simulink model "model_test"  (R2019b)
settings: Solver=VariableStepAuto  StartTime=0.0  StopTime=2000  RelTol=1e-3
values from neighbouring files (symbols this model uses):
  Belt_length = 0.5    [initialization.m]
  n = n+1    (= 2)    [training.m]
  num = 5    [initialization.m]    (also in training.m = 15)
undefined symbols (not defined in the file or in its folder): m, T_product
libraries: simulink x14, sldelib x14, rllib x4
settings Model: Creator=Alexa  LastModifiedBy=Alexa

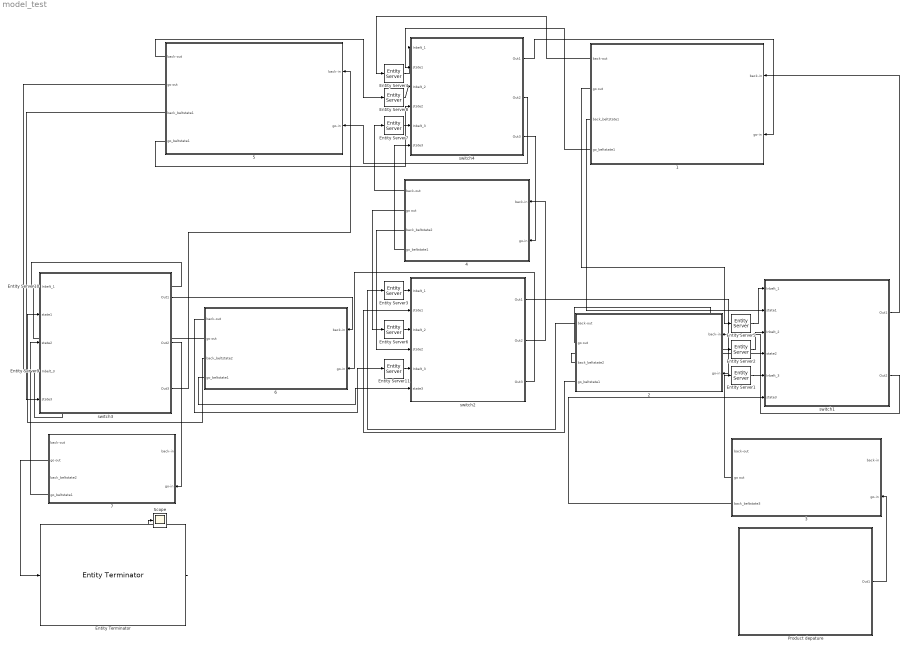
== system model_test ==
  "1 " : Subsystem
      mask Display: image('C:\Users\Alexa\Desktop\MA\writing\pic\thumbnail_image002.jpg'); % Use "Edit Image" on toolstrip to change.
  "2 " : Subsystem
      mask Display: image('C:\Users\Alexa\Desktop\MA\writing\pic\thumbnail_image010.png'); % Use "Edit Image" on toolstrip to change.
  "3 " : Subsystem
      mask Display: image('C:\Users\Alexa\Desktop\MA\writing\pic\thumbnail_image010.png'); % Use "Edit Image" on toolstrip to change.
  4 : Subsystem
      mask Display: image('C:\Users\Alexa\Desktop\MA\writing\pic\thumbnail_image010.png'); % Use "Edit Image" on toolstrip to change.
  5 : Subsystem
      mask Display: image('C:\Users\Alexa\Desktop\MA\writing\pic\thumbnail_image002.jpg'); % Use "Edit Image" on toolstrip to change.
  6 : Subsystem
      mask Display: image('C:\Users\Alexa\Desktop\MA\writing\pic\thumbnail_image010.png'); % Use "Edit Image" on toolstrip to change.
  7 : Subsystem
      mask Display: image('C:\Users\Alexa\Desktop\MA\writing\pic\thumbnail_image010.png'); % Use "Edit Image" on toolstrip to change.
  Entity Server{1,7,9,11} (4 alike) : EntityServer  InputPortMessageModes=m  OutputPortMessageModes=m  Capacity=1  ServiceTimeValue=0  EntryAction=entity.source=3;
  Entity Server{3..5,10} (4 alike) : EntityServer  InputPortMessageModes=m  OutputPortMessageModes=m  Capacity=1  ServiceTimeValue=0  EntryAction=entity.source=1;
  Entity Server2 : EntityServer  InputPortMessageModes=m  OutputPortMessageModes=m  Capacity=1  ServiceTimeValue=0  EntryAction=entity.source=2;
  Entity Server6 : EntityServer  InputPortMessageModes=m  OutputPortMessageModes=m  Capacity=1  ServiceTimeValue=0  EntryAction=entity.source=2;
  Entity Server8 : EntityServer  InputPortMessageModes=m  OutputPortMessageModes=m  Capacity=1  ServiceTimeValue=0  EntryAction=entity.source=2;
  Entity Terminator : EntityTerminator  InputPortMessageModes=m  EntryAction=|  NumberEntitiesArrived=on
      | coder.extrinsic('assignin');
      | persistent Schaltplan;
      | persistent idx;
      | if isempty(Schaltplan)    
      |     idx = 1;
      |     Schaltplan=zeros(2*num+1,1);
      | end
      | Schaltplan(idx)=entity.Record;
      | idx = idx + 1;
      | assignin('base', 'Schaltplan', Schaltplan);
      settings: OutputPortMap=o0
      mask Display: image('C:\Users\Alexa\Desktop\MA\writing\pic\bottle2.JPG'); % Use "Edit Image" on toolstrip to change.
  Product depature : Subsystem
      mask Display: image('C:\Users\Alexa\Desktop\MA\writing\pic\bottle.JPG'); % Use "Edit Image" on toolstrip to change.
  Scope : Scope
  switch1 : Subsystem
      mask Display: image('C:\Users\Alexa\Desktop\MA\writing\pic\thumbnail_image006.jpg'); % Use "Edit Image" on toolstrip to change.
  switch2 : Subsystem
      mask Display: image('C:\Users\Alexa\Desktop\MA\writing\pic\thumbnail_image006.jpg'); % Use "Edit Image" on toolstrip to change.
  switch3 : Subsystem
      mask Display: image('C:\Users\Alexa\Desktop\MA\writing\pic\thumbnail_image006.jpg'); % Use "Edit Image" on toolstrip to change.
  switch4 : Subsystem
      mask Display: image('C:\Users\Alexa\Desktop\MA\writing\pic\thumbnail_image006.jpg'); % Use "Edit Image" on toolstrip to change.
  wires:
  switch1/2(Out2) -> "2 "/1(back-in)
  switch1/1(Out1) -> "1 "/1(back-in)
  "3 "/3(back_beltstate3) -> switch1/6(state3)
  "2 "/3(back_beltstate2) -> switch1/4(state2)
  "1 "/3(back_beltstate1) -> switch1/2(state1)
  Product depature/1(Out1) -> "3 "/2(go-in)
  switch4/1(Out1) -> "1 "/2(go-in)
  Entity Server4/1 -> switch4/1(Inbelt_1)
  "1 "/4(go_beltstate1) -> switch4/2(state1)
  Entity Server5/1 -> switch1/1(Inbelt_1)
  Entity Server2/1 -> switch1/3(Inbelt_2)
  Entity Server1/1 -> switch1/5(Inbelt_3)
  switch2/1(Out1) -> "2 "/2(go-in)
  "2 "/4(go_beltstate1) -> switch2/2(state1)
  Entity Server3/1 -> switch2/1(Inbelt_1)
  Entity Terminator/1 -> Scope/1
  switch4/3(Out3) -> 4/2(go-in)
  switch2/2(Out2) -> 4/1(back-in)
  4/4(go_beltstate1) -> switch4/6(state3)
  4/3(back_beltstate2) -> switch2/4(state2)
  Entity Server6/1 -> switch2/3(Inbelt_2)
  Entity Server7/1 -> switch4/5(Inbelt_3)
  Entity Server8/1 -> switch4/3(Inbelt_2)
  switch4/2(Out2) -> 5/2(go-in)
  5/4(go_beltstate1) -> switch4/4(state2)
  switch3/3(Out3) -> 5/1(back-in)
  5/3(back_beltstate1) -> switch3/5(state3)
  Entity Server9/1 -> switch3/4(Inbelt_3)
  switch2/3(Out3) -> 6/2(go-in)
  Entity Server10/1 -> switch3/1(Inbelt_1)
  6/4(go_beltstate1) -> switch2/6(state3)
  Entity Server11/1 -> switch2/5(Inbelt_3)
  switch3/1(Out1) -> 6/1(back-in)
  6/3(back_beltstate2) -> switch3/2(state1)
  switch3/2(Out2) -> 7/2(go-in)
  7/2(go out) -> Entity Terminator/1
  7/4(go_beltstate1) -> switch3/3(state2)
  "1 "/2(go out) -> Entity Server5/1
  "2 "/2(go out) -> Entity Server2/1
  "3 "/2(go out) -> Entity Server1/1
  "1 "/1(back-out) -> Entity Server4/1
  5/1(back-out) -> Entity Server8/1
  4/1(back-out) -> Entity Server7/1
  "2 "/1(back-out) -> Entity Server3/1
  4/2(go out) -> Entity Server6/1
  6/1(back-out) -> Entity Server11/1
  6/2(go out) -> Entity Server10/1
  5/2(go out) -> Entity Server9/1

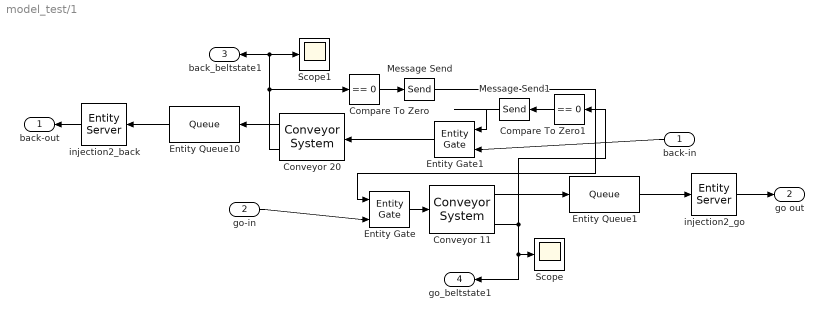
== system model_test/1  ==
  back-in : Inport
  go-in : Inport  Port=2
  Compare To Zero : simulink/Logic and Bit Operations/Compare To Zero  relop===  OutDataTypeStr=boolean
  Compare To Zero1 : simulink/Logic and Bit Operations/Compare To Zero  relop===  OutDataTypeStr=boolean
  Conveyor 11 : sldelib/Conveyor System  mConveyorLength=4*Belt_length  mConveyorSpeedSource=Dialog  mConveyorSpeed=V_belt  mInitialConveyorSpeed=1000  mMinDisBetEntity=Distance_between  mEntityLengthSource=Dialog  mEntityLength=Entity_length  mEntityLengthAttrName=Length  mOutputBlockedOpt=Pause  mErrorUponFullOpt=on  mNumEntitiesDepOpt=on  mNumEntitiesInBlockOpt=on  mEntityPendingOpt=off  mNumExtractedFromBlockOpt=off  mConveyorSpeedOpt=off
      settings: SourceProductName=SimEvents  SourceProductBaseCode=SE
  Conveyor 20 : sldelib/Conveyor System  mConveyorLength=4*Belt_length  mConveyorSpeedSource=Dialog  mConveyorSpeed=V_belt  mInitialConveyorSpeed=1000  mMinDisBetEntity=Distance_between  mEntityLengthSource=Dialog  mEntityLength=Entity_length  mEntityLengthAttrName=Length  mOutputBlockedOpt=Pause  mErrorUponFullOpt=on  mNumEntitiesDepOpt=off  mNumEntitiesInBlockOpt=on  mEntityPendingOpt=off  mNumExtractedFromBlockOpt=off  mConveyorSpeedOpt=off
      settings: SourceProductName=SimEvents  SourceProductBaseCode=SE
  Entity Gate : EntityGate  InputPortMessageModes=m,m  OutputPortMessageModes=m
  Entity Gate1 : EntityGate  InputPortMessageModes=m,m  OutputPortMessageModes=m
  Entity Queue1 : Queue  InputPortMessageModes=m  OutputPortMessageModes=m  Capacity=1
  Entity Queue10 : Queue  InputPortMessageModes=m  OutputPortMessageModes=m  Capacity=1
  Message Send : Send  OutputPortMessageModes=m
  Message Send1 : Send  OutputPortMessageModes=m
  Scope : Scope
  Scope1 : Scope
  injection2_back : EntityServer  InputPortMessageModes=m  OutputPortMessageModes=m  Capacity=1  ServiceTimeSource=Attribute  ServiceTimeAttributeName=Processtime  EntryAction=|
      | if entity.goal==2
      |     entity.finish=1;
      |     entity.Processtime=T_process;
      |     entity.goal=3;
      | else
      |     entity.Processtime=0;
      | end
  injection2_go : EntityServer  InputPortMessageModes=m  OutputPortMessageModes=m  Capacity=1  ServiceTimeSource=Attribute  ServiceTimeAttributeName=Processtime  EntryAction=|
      | if entity.goal==2
      |     entity.finish=1;
      |     entity.Processtime=T_process;
      |     entity.goal=3;
      | else
      |     entity.Processtime=0;
      | end
  back-out : Outport
  go out : Outport  Port=2
  back_beltstate1 : Outport  Port=3
  go_beltstate1 : Outport  Port=4
  wires:
  go-in/1 -> Entity Gate/2
  Conveyor 20/1 -> Entity Queue10/1
  back-in/1 -> Entity Gate1/2
  Compare To Zero1/1 -> Message Send1/1
  Message Send1/1 -> Entity Gate1/1
  Entity Gate1/1 -> Conveyor 20/1
  Conveyor 11/1 -> Entity Queue1/1
  Entity Gate/1 -> Conveyor 11/1
  Compare To Zero/1 -> Message Send/1
  Message Send/1 -> Entity Gate/1
  Conveyor 20/2 -> Compare To Zero/1, Scope1/1, back_beltstate1/1
  Conveyor 11/3 -> go_beltstate1/1, Scope/1, Compare To Zero1/1
  Entity Queue10/1 -> injection2_back/1
  Entity Queue1/1 -> injection2_go/1
  injection2_back/1 -> back-out/1
  injection2_go/1 -> go out/1

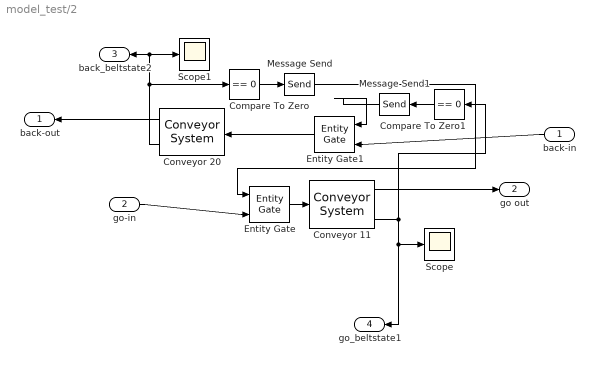
== system model_test/2  ==
  back-in : Inport
  go-in : Inport  Port=2
  Compare To Zero : simulink/Logic and Bit Operations/Compare To Zero  relop===  OutDataTypeStr=boolean
  Compare To Zero1 : simulink/Logic and Bit Operations/Compare To Zero  relop===  OutDataTypeStr=boolean
  Conveyor 11 : sldelib/Conveyor System  mConveyorLength=Belt_length  mConveyorSpeedSource=Dialog  mConveyorSpeed=V_belt  mInitialConveyorSpeed=1000  mMinDisBetEntity=Distance_between  mEntityLengthSource=Dialog  mEntityLength=Entity_length  mEntityLengthAttrName=Length  mOutputBlockedOpt=Pause  mErrorUponFullOpt=on  mNumEntitiesDepOpt=on  mNumEntitiesInBlockOpt=on  mEntityPendingOpt=off  mNumExtractedFromBlockOpt=off  mConveyorSpeedOpt=off
      settings: SourceProductName=SimEvents  SourceProductBaseCode=SE
  Conveyor 20 : sldelib/Conveyor System  mConveyorLength=Belt_length  mConveyorSpeedSource=Dialog  mConveyorSpeed=V_belt  mInitialConveyorSpeed=1000  mMinDisBetEntity=Distance_between  mEntityLengthSource=Dialog  mEntityLength=Entity_length  mEntityLengthAttrName=Length  mOutputBlockedOpt=Pause  mErrorUponFullOpt=on  mNumEntitiesDepOpt=off  mNumEntitiesInBlockOpt=on  mEntityPendingOpt=off  mNumExtractedFromBlockOpt=off  mConveyorSpeedOpt=off
      settings: SourceProductName=SimEvents  SourceProductBaseCode=SE
  Entity Gate : EntityGate  InputPortMessageModes=m,m  OutputPortMessageModes=m
  Entity Gate1 : EntityGate  InputPortMessageModes=m,m  OutputPortMessageModes=m
  Message Send : Send  OutputPortMessageModes=m
  Message Send1 : Send  OutputPortMessageModes=m
  Scope : Scope
  Scope1 : Scope
  back-out : Outport
  go out : Outport  Port=2
  back_beltstate2 : Outport  Port=3
  go_beltstate1 : Outport  Port=4
  wires:
  Conveyor 11/3 -> Compare To Zero1/1, Scope/1, go_beltstate1/1
  Conveyor 20/2 -> Scope1/1, back_beltstate2/1, Compare To Zero/1
  Message Send/1 -> Entity Gate/1
  Compare To Zero/1 -> Message Send/1
  Entity Gate/1 -> Conveyor 11/1
  Conveyor 11/1 -> go out/1
  Entity Gate1/1 -> Conveyor 20/1
  Message Send1/1 -> Entity Gate1/1
  Compare To Zero1/1 -> Message Send1/1
  back-in/1 -> Entity Gate1/2
  Conveyor 20/1 -> back-out/1
  go-in/1 -> Entity Gate/2

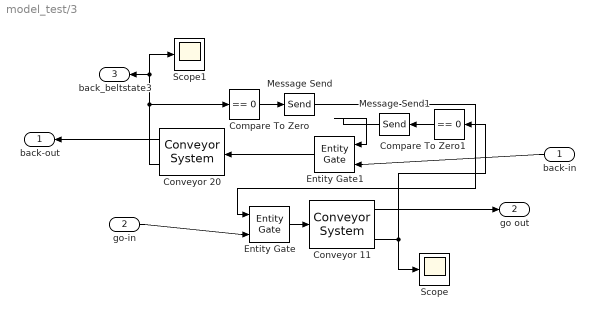
== system model_test/3  ==
  back-in : Inport
  go-in : Inport  Port=2
  Compare To Zero : simulink/Logic and Bit Operations/Compare To Zero  relop===  OutDataTypeStr=boolean
  Compare To Zero1 : simulink/Logic and Bit Operations/Compare To Zero  relop===  OutDataTypeStr=boolean
  Conveyor 11 : sldelib/Conveyor System  mConveyorLength=Belt_length  mConveyorSpeedSource=Dialog  mConveyorSpeed=V_belt  mInitialConveyorSpeed=1000  mMinDisBetEntity=Distance_between  mEntityLengthSource=Dialog  mEntityLength=Entity_length  mEntityLengthAttrName=Length  mOutputBlockedOpt=Pause  mErrorUponFullOpt=on  mNumEntitiesDepOpt=on  mNumEntitiesInBlockOpt=on  mEntityPendingOpt=off  mNumExtractedFromBlockOpt=off  mConveyorSpeedOpt=off
      settings: SourceProductName=SimEvents  SourceProductBaseCode=SE
  Conveyor 20 : sldelib/Conveyor System  mConveyorLength=Belt_length  mConveyorSpeedSource=Dialog  mConveyorSpeed=V_belt  mInitialConveyorSpeed=1000  mMinDisBetEntity=Distance_between  mEntityLengthSource=Dialog  mEntityLength=Entity_length  mEntityLengthAttrName=Length  mOutputBlockedOpt=Pause  mErrorUponFullOpt=on  mNumEntitiesDepOpt=off  mNumEntitiesInBlockOpt=on  mEntityPendingOpt=off  mNumExtractedFromBlockOpt=off  mConveyorSpeedOpt=off
      settings: SourceProductName=SimEvents  SourceProductBaseCode=SE
  Entity Gate : EntityGate  InputPortMessageModes=m,m  OutputPortMessageModes=m
  Entity Gate1 : EntityGate  InputPortMessageModes=m,m  OutputPortMessageModes=m
  Message Send : Send  OutputPortMessageModes=m
  Message Send1 : Send  OutputPortMessageModes=m
  Scope : Scope
  Scope1 : Scope
  back-out : Outport
  go out : Outport  Port=2
  back_beltstate3 : Outport  Port=3
  wires:
  Conveyor 11/3 -> Scope/1, Compare To Zero1/1
  Conveyor 20/2 -> Scope1/1, back_beltstate3/1, Compare To Zero/1
  Message Send/1 -> Entity Gate/1
  Compare To Zero/1 -> Message Send/1
  Entity Gate/1 -> Conveyor 11/1
  Conveyor 11/1 -> go out/1
  Entity Gate1/1 -> Conveyor 20/1
  Message Send1/1 -> Entity Gate1/1
  Compare To Zero1/1 -> Message Send1/1
  back-in/1 -> Entity Gate1/2
  Conveyor 20/1 -> back-out/1
  go-in/1 -> Entity Gate/2

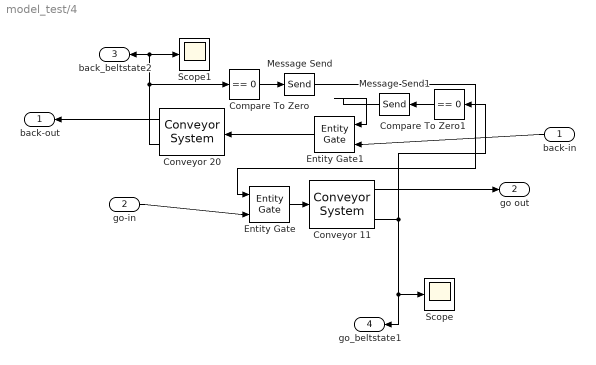
== system model_test/4 ==
  back-in : Inport
  go-in : Inport  Port=2
  Compare To Zero : simulink/Logic and Bit Operations/Compare To Zero  relop===  OutDataTypeStr=boolean
  Compare To Zero1 : simulink/Logic and Bit Operations/Compare To Zero  relop===  OutDataTypeStr=boolean
  Conveyor 11 : sldelib/Conveyor System  mConveyorLength=Belt_length  mConveyorSpeedSource=Dialog  mConveyorSpeed=V_belt  mInitialConveyorSpeed=1000  mMinDisBetEntity=Distance_between  mEntityLengthSource=Dialog  mEntityLength=Entity_length  mEntityLengthAttrName=Length  mOutputBlockedOpt=Pause  mErrorUponFullOpt=on  mNumEntitiesDepOpt=on  mNumEntitiesInBlockOpt=on  mEntityPendingOpt=off  mNumExtractedFromBlockOpt=off  mConveyorSpeedOpt=off
      settings: SourceProductName=SimEvents  SourceProductBaseCode=SE
  Conveyor 20 : sldelib/Conveyor System  mConveyorLength=Belt_length  mConveyorSpeedSource=Dialog  mConveyorSpeed=V_belt  mInitialConveyorSpeed=1000  mMinDisBetEntity=Distance_between  mEntityLengthSource=Dialog  mEntityLength=Entity_length  mEntityLengthAttrName=Length  mOutputBlockedOpt=Pause  mErrorUponFullOpt=on  mNumEntitiesDepOpt=off  mNumEntitiesInBlockOpt=on  mEntityPendingOpt=off  mNumExtractedFromBlockOpt=off  mConveyorSpeedOpt=off
      settings: SourceProductName=SimEvents  SourceProductBaseCode=SE
  Entity Gate : EntityGate  InputPortMessageModes=m,m  OutputPortMessageModes=m
  Entity Gate1 : EntityGate  InputPortMessageModes=m,m  OutputPortMessageModes=m
  Message Send : Send  OutputPortMessageModes=m
  Message Send1 : Send  OutputPortMessageModes=m
  Scope : Scope
  Scope1 : Scope
  back-out : Outport
  go out : Outport  Port=2
  back_beltstate2 : Outport  Port=3
  go_beltstate1 : Outport  Port=4
  wires:
  go-in/1 -> Entity Gate/2
  Conveyor 20/1 -> back-out/1
  back-in/1 -> Entity Gate1/2
  Compare To Zero1/1 -> Message Send1/1
  Message Send1/1 -> Entity Gate1/1
  Entity Gate1/1 -> Conveyor 20/1
  Conveyor 11/1 -> go out/1
  Entity Gate/1 -> Conveyor 11/1
  Compare To Zero/1 -> Message Send/1
  Message Send/1 -> Entity Gate/1
  Conveyor 20/2 -> Compare To Zero/1, Scope1/1, back_beltstate2/1
  Conveyor 11/3 -> go_beltstate1/1, Scope/1, Compare To Zero1/1

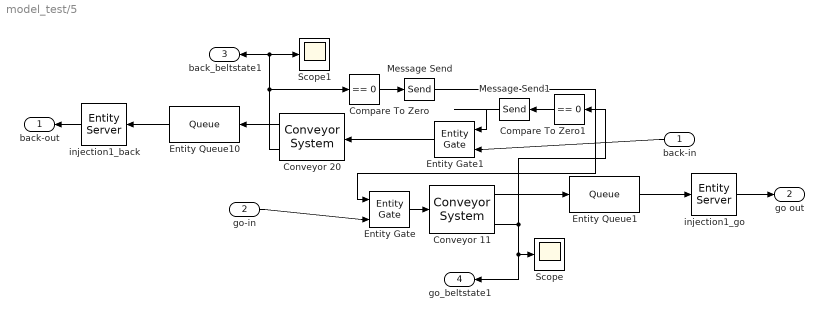
== system model_test/5 ==
  back-in : Inport
  go-in : Inport  Port=2
  Compare To Zero : simulink/Logic and Bit Operations/Compare To Zero  relop===  OutDataTypeStr=boolean
  Compare To Zero1 : simulink/Logic and Bit Operations/Compare To Zero  relop===  OutDataTypeStr=boolean
  Conveyor 11 : sldelib/Conveyor System  mConveyorLength=4*Belt_length  mConveyorSpeedSource=Dialog  mConveyorSpeed=V_belt  mInitialConveyorSpeed=1000  mMinDisBetEntity=Distance_between  mEntityLengthSource=Dialog  mEntityLength=Entity_length  mEntityLengthAttrName=Length  mOutputBlockedOpt=Pause  mErrorUponFullOpt=on  mNumEntitiesDepOpt=on  mNumEntitiesInBlockOpt=on  mEntityPendingOpt=off  mNumExtractedFromBlockOpt=off  mConveyorSpeedOpt=off
      settings: SourceProductName=SimEvents  SourceProductBaseCode=SE
  Conveyor 20 : sldelib/Conveyor System  mConveyorLength=4*Belt_length  mConveyorSpeedSource=Dialog  mConveyorSpeed=V_belt  mInitialConveyorSpeed=1000  mMinDisBetEntity=Distance_between  mEntityLengthSource=Dialog  mEntityLength=Entity_length  mEntityLengthAttrName=Length  mOutputBlockedOpt=Pause  mErrorUponFullOpt=on  mNumEntitiesDepOpt=off  mNumEntitiesInBlockOpt=on  mEntityPendingOpt=off  mNumExtractedFromBlockOpt=off  mConveyorSpeedOpt=off
      settings: SourceProductName=SimEvents  SourceProductBaseCode=SE
  Entity Gate : EntityGate  InputPortMessageModes=m,m  OutputPortMessageModes=m
  Entity Gate1 : EntityGate  InputPortMessageModes=m,m  OutputPortMessageModes=m
  Entity Queue1 : Queue  InputPortMessageModes=m  OutputPortMessageModes=m  Capacity=1
  Entity Queue10 : Queue  InputPortMessageModes=m  OutputPortMessageModes=m  Capacity=1
  Message Send : Send  OutputPortMessageModes=m
  Message Send1 : Send  OutputPortMessageModes=m
  Scope : Scope
  Scope1 : Scope
  injection1_back : EntityServer  InputPortMessageModes=m  OutputPortMessageModes=m  Capacity=1  ServiceTimeSource=Attribute  ServiceTimeAttributeName=Processtime  EntryAction=|
      | if entity.goal==1
      |     entity.finish=1;
      |     entity.Processtime=T_process;
      |     entity.goal=3;
      | else
      |     entity.Processtime=0;
      | end
  injection1_go : EntityServer  InputPortMessageModes=m  OutputPortMessageModes=m  Capacity=1  ServiceTimeSource=Attribute  ServiceTimeAttributeName=Processtime  EntryAction=|
      | if entity.goal==1
      |     entity.finish=1;
      |     entity.Processtime=T_process;
      |     entity.goal=3;
      | else
      |     entity.Processtime=0;
      | end
  back-out : Outport
  go out : Outport  Port=2
  back_beltstate1 : Outport  Port=3
  go_beltstate1 : Outport  Port=4
  wires:
  injection1_go/1 -> go out/1
  injection1_back/1 -> back-out/1
  Entity Queue1/1 -> injection1_go/1
  Entity Queue10/1 -> injection1_back/1
  Conveyor 11/3 -> Compare To Zero1/1, go_beltstate1/1, Scope/1
  Conveyor 20/2 -> back_beltstate1/1, Scope1/1, Compare To Zero/1
  Message Send/1 -> Entity Gate/1
  Compare To Zero/1 -> Message Send/1
  Entity Gate/1 -> Conveyor 11/1
  Conveyor 11/1 -> Entity Queue1/1
  Entity Gate1/1 -> Conveyor 20/1
  Message Send1/1 -> Entity Gate1/1
  Compare To Zero1/1 -> Message Send1/1
  back-in/1 -> Entity Gate1/2
  Conveyor 20/1 -> Entity Queue10/1
  go-in/1 -> Entity Gate/2

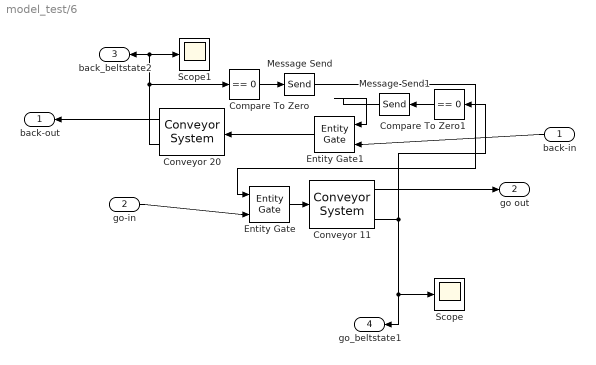
== system model_test/6 ==
  back-in : Inport
  go-in : Inport  Port=2
  Compare To Zero : simulink/Logic and Bit Operations/Compare To Zero  relop===  OutDataTypeStr=boolean
  Compare To Zero1 : simulink/Logic and Bit Operations/Compare To Zero  relop===  OutDataTypeStr=boolean
  Conveyor 11 : sldelib/Conveyor System  mConveyorLength=Belt_length  mConveyorSpeedSource=Dialog  mConveyorSpeed=V_belt  mInitialConveyorSpeed=1000  mMinDisBetEntity=Distance_between  mEntityLengthSource=Dialog  mEntityLength=Entity_length  mEntityLengthAttrName=Length  mOutputBlockedOpt=Pause  mErrorUponFullOpt=on  mNumEntitiesDepOpt=on  mNumEntitiesInBlockOpt=on  mEntityPendingOpt=off  mNumExtractedFromBlockOpt=off  mConveyorSpeedOpt=off
      settings: SourceProductName=SimEvents  SourceProductBaseCode=SE
  Conveyor 20 : sldelib/Conveyor System  mConveyorLength=Belt_length  mConveyorSpeedSource=Dialog  mConveyorSpeed=V_belt  mInitialConveyorSpeed=1000  mMinDisBetEntity=Distance_between  mEntityLengthSource=Dialog  mEntityLength=Entity_length  mEntityLengthAttrName=Length  mOutputBlockedOpt=Pause  mErrorUponFullOpt=on  mNumEntitiesDepOpt=off  mNumEntitiesInBlockOpt=on  mEntityPendingOpt=off  mNumExtractedFromBlockOpt=off  mConveyorSpeedOpt=off
      settings: SourceProductName=SimEvents  SourceProductBaseCode=SE
  Entity Gate : EntityGate  InputPortMessageModes=m,m  OutputPortMessageModes=m
  Entity Gate1 : EntityGate  InputPortMessageModes=m,m  OutputPortMessageModes=m
  Message Send : Send  OutputPortMessageModes=m
  Message Send1 : Send  OutputPortMessageModes=m
  Scope : Scope
  Scope1 : Scope
  back-out : Outport
  go out : Outport  Port=2
  back_beltstate2 : Outport  Port=3
  go_beltstate1 : Outport  Port=4
  wires:
  Conveyor 11/3 -> Compare To Zero1/1, go_beltstate1/1, Scope/1
  Conveyor 20/2 -> Scope1/1, back_beltstate2/1, Compare To Zero/1
  Message Send/1 -> Entity Gate/1
  Compare To Zero/1 -> Message Send/1
  Entity Gate/1 -> Conveyor 11/1
  Conveyor 11/1 -> go out/1
  Entity Gate1/1 -> Conveyor 20/1
  Message Send1/1 -> Entity Gate1/1
  Compare To Zero1/1 -> Message Send1/1
  back-in/1 -> Entity Gate1/2
  Conveyor 20/1 -> back-out/1
  go-in/1 -> Entity Gate/2

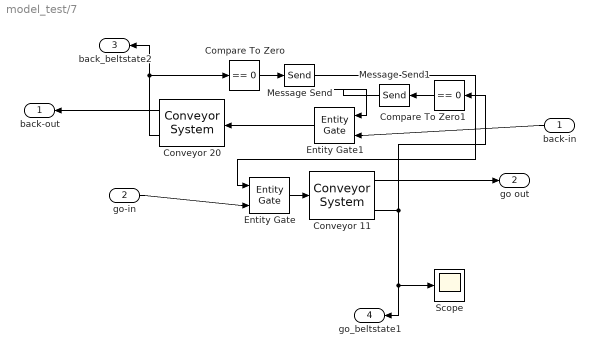
== system model_test/7 ==
  back-in : Inport
  go-in : Inport  Port=2
  Compare To Zero : simulink/Logic and Bit Operations/Compare To Zero  relop===  OutDataTypeStr=boolean
  Compare To Zero1 : simulink/Logic and Bit Operations/Compare To Zero  relop===  OutDataTypeStr=boolean
  Conveyor 11 : sldelib/Conveyor System  mConveyorLength=Belt_length  mConveyorSpeedSource=Dialog  mConveyorSpeed=V_belt  mInitialConveyorSpeed=1000  mMinDisBetEntity=Distance_between  mEntityLengthSource=Dialog  mEntityLength=Entity_length  mEntityLengthAttrName=Length  mOutputBlockedOpt=Pause  mErrorUponFullOpt=on  mNumEntitiesDepOpt=on  mNumEntitiesInBlockOpt=on  mEntityPendingOpt=off  mNumExtractedFromBlockOpt=off  mConveyorSpeedOpt=off
      settings: SourceProductName=SimEvents  SourceProductBaseCode=SE
  Conveyor 20 : sldelib/Conveyor System  mConveyorLength=Belt_length  mConveyorSpeedSource=Dialog  mConveyorSpeed=V_belt  mInitialConveyorSpeed=1000  mMinDisBetEntity=Distance_between  mEntityLengthSource=Dialog  mEntityLength=Entity_length  mEntityLengthAttrName=Length  mOutputBlockedOpt=Pause  mErrorUponFullOpt=on  mNumEntitiesDepOpt=off  mNumEntitiesInBlockOpt=on  mEntityPendingOpt=off  mNumExtractedFromBlockOpt=off  mConveyorSpeedOpt=off
      settings: SourceProductName=SimEvents  SourceProductBaseCode=SE
  Entity Gate : EntityGate  InputPortMessageModes=m,m  OutputPortMessageModes=m
  Entity Gate1 : EntityGate  InputPortMessageModes=m,m  OutputPortMessageModes=m
  Message Send : Send  OutputPortMessageModes=m
  Message Send1 : Send  OutputPortMessageModes=m
  Scope : Scope
  back-out : Outport
  go out : Outport  Port=2
  back_beltstate2 : Outport  Port=3
  go_beltstate1 : Outport  Port=4
  wires:
  go-in/1 -> Entity Gate/2
  Conveyor 20/1 -> back-out/1
  back-in/1 -> Entity Gate1/2
  Compare To Zero1/1 -> Message Send1/1
  Message Send1/1 -> Entity Gate1/1
  Entity Gate1/1 -> Conveyor 20/1
  Conveyor 11/1 -> go out/1
  Entity Gate/1 -> Conveyor 11/1
  Compare To Zero/1 -> Message Send/1
  Message Send/1 -> Entity Gate/1
  Conveyor 20/2 -> Compare To Zero/1, back_beltstate2/1
  Conveyor 11/3 -> go_beltstate1/1, Scope/1, Compare To Zero1/1

== system model_test/Product depature ==
  Abs : Abs
  Abs1 : Abs
  Entity Input Switch : EntityInputSwitch  InputPortMessageModes=m,m  OutputPortMessageModes=m
  Mux1 : Mux  Inputs=2
  Scope1 : Scope
  input entrance1 : EntityGenerator  OutputPortMessageModes=n,m  TimeSource=MATLAB action  Period=T_product  IntergenerationTimeAction=|  AttributeName=Record|Processtime|finish|goal|source  AttributeInitialValue=1|T_process|0|1|0  NumberEntitiesDeparted=on  EntityType=Structured  EntityTypeName=Entity
      | % Pattern: Repeating Sequence
      | persistent idx1;
      | if isempty(idx1)
      |     idx1 = 1;
      | end
      | if idx1 > num-1
      |     dt = inf;
      | else
      | %    dt = T_interval;
      |     dt = 2*T_interval;
      | end
      | idx1 = idx1 + 1;
      settings: OutputPortMap=o0,o3
  input entrance2 : EntityGenerator  OutputPortMessageModes=n,m  TimeSource=MATLAB action  Period=T_product  IntergenerationTimeAction=|  GenerateEntityAtSimulationStart=off  AttributeName=Record|Processtime|finish|goal|source  AttributeInitialValue=1|T_process|0|2|0  NumberEntitiesDeparted=on  EntityType=Structured  EntityTypeName=Entity
      | % Pattern: Repeating Sequence
      | persistent idx1;
      | if isempty(idx1)
      |     idx1 = 1;
      | end
      | if idx1==1
      | %    dt = 500;
      |     dt =T_interval;
      | elseif idx1 > num
      |     dt = inf;
      | else
      | %    dt = T_interval;
      |     dt =2*T_interval;
      | end
      | idx1 = idx1 + 1;
      settings: OutputPortMap=o0,o3
  Out1 : Outport
  wires:
  Entity Input Switch/1 -> Out1/1
  input entrance2/2 -> Entity Input Switch/2
  input entrance1/2 -> Entity Input Switch/1
  input entrance1/1 -> Abs/1
  input entrance2/1 -> Abs1/1
  Abs/1 -> Mux1/1
  Abs1/1 -> Mux1/2
  Mux1/1 -> Scope1/1

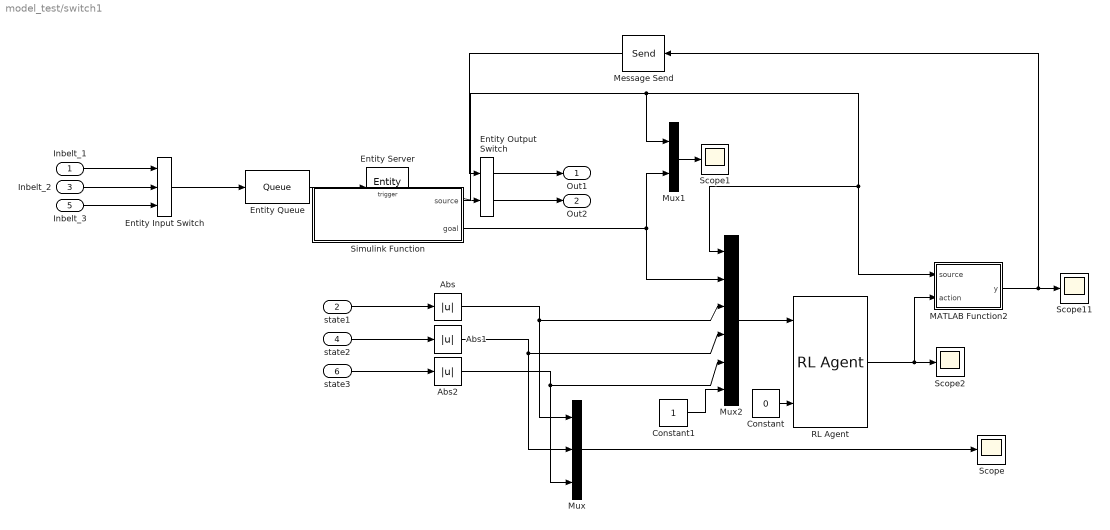
== system model_test/switch1 ==
  Inbelt_1 : Inport
  state1 : Inport  Port=2
  Inbelt_2 : Inport  Port=3
  state2 : Inport  Port=4
  Inbelt_3 : Inport  Port=5
  state3 : Inport  Port=6
  Abs : Abs
  Abs1 : Abs
  Abs2 : Abs
  Constant : Constant  Value=0
  Constant1 : Constant
  Entity Input Switch : EntityInputSwitch  InputPortMessageModes=m,m,m  OutputPortMessageModes=m  NumberInputPorts=3
      settings: InputPortMap=u1,u2,u3
  Entity Output Switch : EntityOutputSwitch  InputPortMessageModes=m,m  OutputPortMessageModes=m,m  SwitchingCriterion=From control port  SwitchAttributeName=Attribute1
      settings: InputPortMap=u0,u1
  Entity Queue : Queue  InputPortMessageModes=m  OutputPortMessageModes=m  Capacity=2*num
  Entity Server : EntityServer  InputPortMessageModes=m  OutputPortMessageModes=m  Capacity=1  ServiceTimeValue=T_switch  EntryAction=|
      | getattribute1(entity.source,entity.goal);
      | entity.Record = entity.Record*10+1;
  MATLAB Function2 : MATLAB Function  TreatAsAtomicUnit=on
  Message Send : Send  OutputPortMessageModes=m
  Mux : Mux  Inputs=3
  Mux1 : Mux  Inputs=2
  Mux2 : Mux  Inputs=6
  RL Agent : rllib/RL Agent  Agent=agent  ProvideReward=on  ProvideIsDone=on  ProvideCumRwd=off  TreatAsDirectFeedthrough=on  CollectLoggedSignals=on  CollectModelStates=on
      settings: SourceProductName=Reinforcement Learning Toolbox
  Scope{,1..2,11} (4 alike) : Scope
  Simulink Function : Subsystem  TreatAsAtomicUnit=on
  Out1 : Outport
  Out2 : Outport  Port=2
  wires:
  Entity Server/1 -> Entity Output Switch/2
  Abs/1 -> Mux2/3, Mux/1
  Abs1/1 -> Mux2/4, Mux/2
  Mux1/1 -> Scope1/1
  Simulink Function/2(goal) -> Mux2/2, Mux1/2
  state1/1 -> Abs/1
  MATLAB Function2/1(y) -> Message Send/1, Scope11/1
  Entity Queue/1 -> Entity Server/1
  Simulink Function/1(source) -> Mux2/1, MATLAB Function2/1(source), Mux1/1
  RL Agent/1 -> MATLAB Function2/2(action), Scope2/1
  Entity Output Switch/1 -> Out1/1
  Entity Output Switch/2 -> Out2/1
  Entity Input Switch/1 -> Entity Queue/1
  Abs2/1 -> Mux2/5, Mux/3
  Mux/1 -> Scope/1
  Inbelt_3/1 -> Entity Input Switch/3
  state3/1 -> Abs2/1
  Constant/1 -> RL Agent/3
  Message Send/1 -> Entity Output Switch/1
  Mux2/1 -> RL Agent/1
  Inbelt_2/1 -> Entity Input Switch/2
  Inbelt_1/1 -> Entity Input Switch/1
  state2/1 -> Abs1/1
  Constant1/1 -> Mux2/6

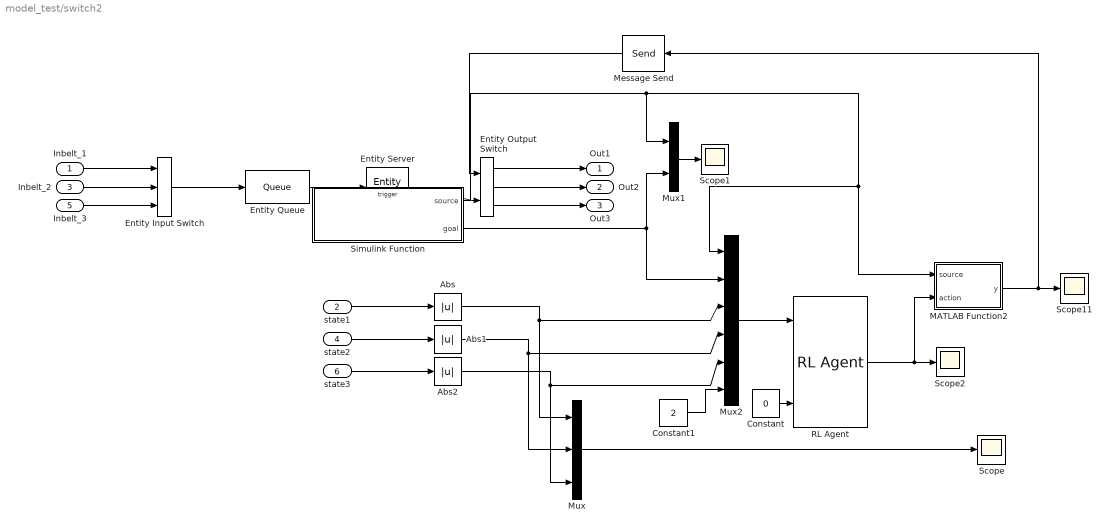
== system model_test/switch2 ==
  Inbelt_1 : Inport
  state1 : Inport  Port=2
  Inbelt_2 : Inport  Port=3
  state2 : Inport  Port=4
  Inbelt_3 : Inport  Port=5
  state3 : Inport  Port=6
  Abs : Abs
  Abs1 : Abs
  Abs2 : Abs
  Constant : Constant  Value=0
  Constant1 : Constant  Value=2
  Entity Input Switch : EntityInputSwitch  InputPortMessageModes=m,m,m  OutputPortMessageModes=m  NumberInputPorts=3
      settings: InputPortMap=u1,u2,u3
  Entity Output Switch : EntityOutputSwitch  InputPortMessageModes=m,m  OutputPortMessageModes=m,m,m  NumberOutputPorts=3  SwitchingCriterion=From control port  SwitchAttributeName=Attribute1
      settings: InputPortMap=u0,u1  OutputPortMap=o0,o1,o2
  Entity Queue : Queue  InputPortMessageModes=m  OutputPortMessageModes=m  Capacity=2*num
  Entity Server : EntityServer  InputPortMessageModes=m  OutputPortMessageModes=m  Capacity=1  ServiceTimeValue=T_switch  EntryAction=|
      | getattribute2(entity.source,entity.goal);
      | entity.Record = entity.Record*10+2;
  MATLAB Function2 : MATLAB Function  TreatAsAtomicUnit=on
  Message Send : Send  OutputPortMessageModes=m
  Mux : Mux  Inputs=3
  Mux1 : Mux  Inputs=2
  Mux2 : Mux  Inputs=6
  RL Agent : rllib/RL Agent  Agent=agent  ProvideReward=on  ProvideIsDone=on  ProvideCumRwd=off  TreatAsDirectFeedthrough=on  CollectLoggedSignals=on  CollectModelStates=on
      settings: SourceProductName=Reinforcement Learning Toolbox
  Scope{,1..2,11} (4 alike) : Scope
  Simulink Function : Subsystem  TreatAsAtomicUnit=on
  Out1 : Outport
  Out2 : Outport  Port=2
  Out3 : Outport  Port=3
  wires:
  state2/1 -> Abs1/1
  Inbelt_1/1 -> Entity Input Switch/1
  Inbelt_2/1 -> Entity Input Switch/2
  Mux2/1 -> RL Agent/1
  Message Send/1 -> Entity Output Switch/1
  Entity Output Switch/3 -> Out3/1
  Constant/1 -> RL Agent/3
  state3/1 -> Abs2/1
  Inbelt_3/1 -> Entity Input Switch/3
  Mux/1 -> Scope/1
  Abs2/1 -> Mux/3, Mux2/5
  Entity Input Switch/1 -> Entity Queue/1
  Entity Output Switch/2 -> Out2/1
  Entity Output Switch/1 -> Out1/1
  RL Agent/1 -> Scope2/1, MATLAB Function2/2(action)
  Simulink Function/1(source) -> Mux1/1, MATLAB Function2/1(source), Mux2/1
  Entity Queue/1 -> Entity Server/1
  MATLAB Function2/1(y) -> Scope11/1, Message Send/1
  state1/1 -> Abs/1
  Simulink Function/2(goal) -> Mux1/2, Mux2/2
  Mux1/1 -> Scope1/1
  Abs1/1 -> Mux/2, Mux2/4
  Abs/1 -> Mux/1, Mux2/3
  Entity Server/1 -> Entity Output Switch/2
  Constant1/1 -> Mux2/6

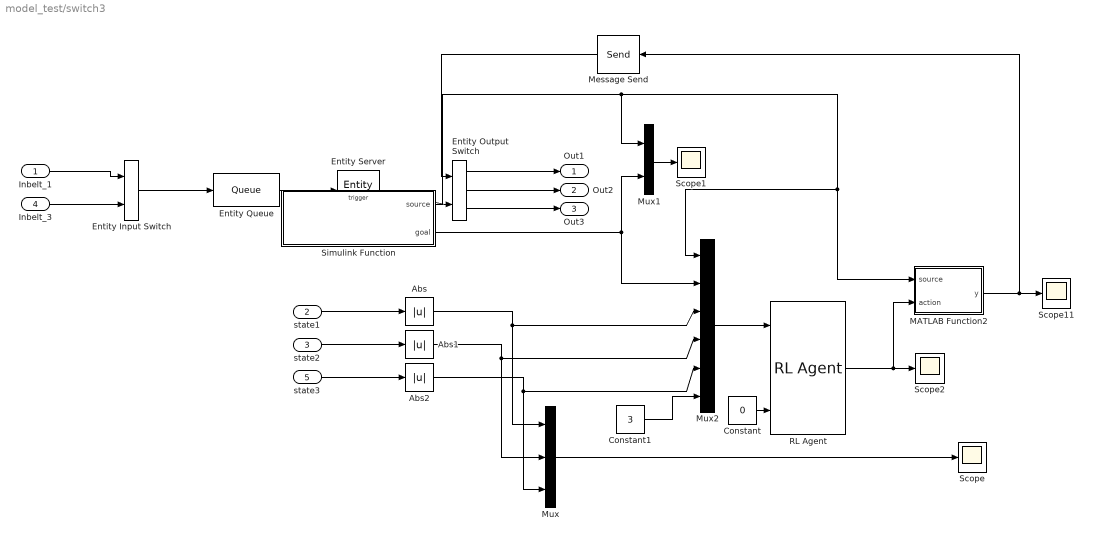
== system model_test/switch3 ==
  Inbelt_1 : Inport
  state1 : Inport  Port=2
  state2 : Inport  Port=3
  Inbelt_3 : Inport  Port=4
  state3 : Inport  Port=5
  Abs : Abs
  Abs1 : Abs
  Abs2 : Abs
  Constant : Constant  Value=0
  Constant1 : Constant  Value=3
  Entity Input Switch : EntityInputSwitch  InputPortMessageModes=m,m  OutputPortMessageModes=m
  Entity Output Switch : EntityOutputSwitch  InputPortMessageModes=m,m  OutputPortMessageModes=m,m,m  NumberOutputPorts=3  SwitchingCriterion=From control port  SwitchAttributeName=Attribute1
      settings: InputPortMap=u0,u1  OutputPortMap=o0,o1,o2
  Entity Queue : Queue  InputPortMessageModes=m  OutputPortMessageModes=m  Capacity=2*num
  Entity Server : EntityServer  InputPortMessageModes=m  OutputPortMessageModes=m  Capacity=1  ServiceTimeValue=T_switch  EntryAction=|
      | getattribute3(entity.source,entity.goal);
      | entity.Record = entity.Record*10+3;
  MATLAB Function2 : MATLAB Function  TreatAsAtomicUnit=on
  Message Send : Send  OutputPortMessageModes=m
  Mux : Mux  Inputs=3
  Mux1 : Mux  Inputs=2
  Mux2 : Mux  Inputs=6
  RL Agent : rllib/RL Agent  Agent=agent  ProvideReward=on  ProvideIsDone=on  ProvideCumRwd=off  TreatAsDirectFeedthrough=on  CollectLoggedSignals=on  CollectModelStates=on
      settings: SourceProductName=Reinforcement Learning Toolbox
  Scope{,1..2,11} (4 alike) : Scope
  Simulink Function : Subsystem  TreatAsAtomicUnit=on
  Out1 : Outport
  Out2 : Outport  Port=2
  Out3 : Outport  Port=3
  wires:
  Entity Server/1 -> Entity Output Switch/2
  Abs/1 -> Mux2/3, Mux/1
  Abs1/1 -> Mux2/4, Mux/2
  Mux1/1 -> Scope1/1
  Simulink Function/2(goal) -> Mux2/2, Mux1/2
  state1/1 -> Abs/1
  MATLAB Function2/1(y) -> Message Send/1, Scope11/1
  Entity Queue/1 -> Entity Server/1
  Simulink Function/1(source) -> Mux2/1, MATLAB Function2/1(source), Mux1/1
  RL Agent/1 -> MATLAB Function2/2(action), Scope2/1
  Entity Output Switch/1 -> Out1/1
  Entity Output Switch/2 -> Out2/1
  Entity Input Switch/1 -> Entity Queue/1
  Abs2/1 -> Mux2/5, Mux/3
  Mux/1 -> Scope/1
  state3/1 -> Abs2/1
  Constant/1 -> RL Agent/3
  Entity Output Switch/3 -> Out3/1
  Message Send/1 -> Entity Output Switch/1
  Mux2/1 -> RL Agent/1
  Inbelt_1/1 -> Entity Input Switch/1
  state2/1 -> Abs1/1
  Inbelt_3/1 -> Entity Input Switch/2
  Constant1/1 -> Mux2/6

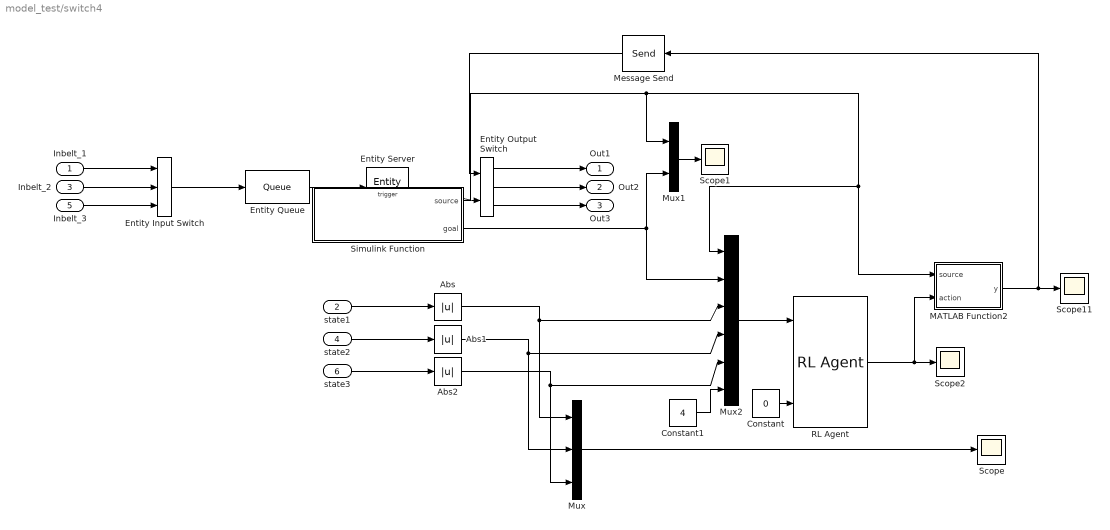
== system model_test/switch4 ==
  Inbelt_1 : Inport
  state1 : Inport  Port=2
  Inbelt_2 : Inport  Port=3
  state2 : Inport  Port=4
  Inbelt_3 : Inport  Port=5
  state3 : Inport  Port=6
  Abs : Abs
  Abs1 : Abs
  Abs2 : Abs
  Constant : Constant  Value=0
  Constant1 : Constant  Value=4
  Entity Input Switch : EntityInputSwitch  InputPortMessageModes=m,m,m  OutputPortMessageModes=m  NumberInputPorts=3
      settings: InputPortMap=u1,u2,u3
  Entity Output Switch : EntityOutputSwitch  InputPortMessageModes=m,m  OutputPortMessageModes=m,m,m  NumberOutputPorts=3  SwitchingCriterion=From control port  SwitchAttributeName=Attribute1
      settings: InputPortMap=u0,u1  OutputPortMap=o0,o1,o2
  Entity Queue : Queue  InputPortMessageModes=m  OutputPortMessageModes=m  Capacity=2*num
  Entity Server : EntityServer  InputPortMessageModes=m  OutputPortMessageModes=m  Capacity=1  ServiceTimeValue=T_switch  EntryAction=|
      | getattribute4(entity.source,entity.goal);
      | entity.Record = entity.Record*10+4;
  MATLAB Function2 : MATLAB Function  TreatAsAtomicUnit=on
  Message Send : Send  OutputPortMessageModes=m
  Mux : Mux  Inputs=3
  Mux1 : Mux  Inputs=2
  Mux2 : Mux  Inputs=6
  RL Agent : rllib/RL Agent  Agent=agent  ProvideReward=on  ProvideIsDone=on  ProvideCumRwd=off  TreatAsDirectFeedthrough=on  CollectLoggedSignals=on  CollectModelStates=on
      settings: SourceProductName=Reinforcement Learning Toolbox
  Scope{,1..2,11} (4 alike) : Scope
  Simulink Function : Subsystem  TreatAsAtomicUnit=on
  Out1 : Outport
  Out2 : Outport  Port=2
  Out3 : Outport  Port=3
  wires:
  state2/1 -> Abs1/1
  Inbelt_1/1 -> Entity Input Switch/1
  Inbelt_2/1 -> Entity Input Switch/2
  Mux2/1 -> RL Agent/1
  Message Send/1 -> Entity Output Switch/1
  Entity Output Switch/3 -> Out3/1
  Constant/1 -> RL Agent/3
  state3/1 -> Abs2/1
  Inbelt_3/1 -> Entity Input Switch/3
  Mux/1 -> Scope/1
  Abs2/1 -> Mux/3, Mux2/5
  Entity Input Switch/1 -> Entity Queue/1
  Entity Output Switch/2 -> Out2/1
  Entity Output Switch/1 -> Out1/1
  RL Agent/1 -> Scope2/1, MATLAB Function2/2(action)
  Simulink Function/1(source) -> Mux1/1, MATLAB Function2/1(source), Mux2/1
  Entity Queue/1 -> Entity Server/1
  MATLAB Function2/1(y) -> Scope11/1, Message Send/1
  state1/1 -> Abs/1
  Simulink Function/2(goal) -> Mux1/2, Mux2/2
  Mux1/1 -> Scope1/1
  Abs1/1 -> Mux/2, Mux2/4
  Abs/1 -> Mux/1, Mux2/3
  Entity Server/1 -> Entity Output Switch/2
  Constant1/1 -> Mux2/6

== system model_test/switch1/Simulink Function ==
  f : TriggerPort  TriggerType=function-call  IsSimulinkFunction=on  FunctionName=getattribute1  VariantControl=(inherit)
  entity : ArgIn  DisableCoverage=on  ArgumentName=source
  entity1 : ArgIn  DisableCoverage=on  Port=2  ArgumentName=goal
  source : Outport
  goal : Outport  Port=2
  wires:
  entity/1 -> source/1
  entity1/1 -> goal/1

== system model_test/switch2/Simulink Function ==
  f : TriggerPort  TriggerType=function-call  IsSimulinkFunction=on  FunctionName=getattribute2  VariantControl=(inherit)
  entity : ArgIn  DisableCoverage=on  ArgumentName=source
  entity1 : ArgIn  DisableCoverage=on  Port=2  ArgumentName=goal
  source : Outport
  goal : Outport  Port=2
  wires:
  entity1/1 -> goal/1
  entity/1 -> source/1

== system model_test/switch3/Simulink Function ==
  f : TriggerPort  TriggerType=function-call  IsSimulinkFunction=on  FunctionName=getattribute3  VariantControl=(inherit)
  entity : ArgIn  DisableCoverage=on  ArgumentName=source
  entity1 : ArgIn  DisableCoverage=on  Port=2  ArgumentName=goal
  source : Outport
  goal : Outport  Port=2
  wires:
  entity/1 -> source/1
  entity1/1 -> goal/1

== system model_test/switch4/Simulink Function ==
  f : TriggerPort  TriggerType=function-call  IsSimulinkFunction=on  FunctionName=getattribute4  VariantControl=(inherit)
  entity : ArgIn  DisableCoverage=on  ArgumentName=source
  entity1 : ArgIn  DisableCoverage=on  Port=2  ArgumentName=goal
  source : Outport
  goal : Outport  Port=2
  wires:
  entity1/1 -> goal/1
  entity/1 -> source/1

== matlab function model_test/switch4/MATLAB Function2 ==
  data: source input; y output; action input
function y = fcn(source,action)
if source==1
    if action==1
        y=2;
    else
        y=3;
    end
elseif source==2
     if action==1
        y=1;
    else
        y=3;
    end
elseif source==3
     if action==1
        y=1;
    else
        y=2;
     end
else
    y=1;
end
end

== matlab function model_test/switch2/MATLAB Function2 ==
  data: source input; y output; action input
function y = fcn(source,action)
if source==1
    if action==1
        y=2;
    else
        y=3;
    end
elseif source==2
     if action==1
        y=1;
    else
        y=3;
    end
elseif source==3
     if action==1
        y=1;
    else
        y=2;
     end
else
    y=1;
end
end

== matlab function model_test/switch3/MATLAB Function2 ==
  data: source input; y output; action input
function y = fcn(source,action)
if source==1
    if action==1
        y=2;
    else
        y=3;
    end
elseif source==2
     if action==1
        y=1;
    else
        y=3;
    end
elseif source==3
     if action==1
        y=1;
    else
        y=2;
     end
else
    y=1;
end
end

== matlab function model_test/switch1/MATLAB Function2 ==
  data: source input; y output; action input
function y = fcn(source,action)
%% switch_1
if source==1
    y=2;
elseif source==2
    y=1;
else
    if action==1
        y=1;
    else
        y=2;
    end
end
end
